simulink model "model_ciagly"  (R2019b)
settings: Solver=FixedStepAuto  StartTime=0  StopTime=4  FixedStep=0.0002  RelTol=1e-3
values from neighbouring files (symbols this model uses):
  J = 22*Js    (= 6.05)    [P.m]    (also in PI.m; faza.m)
  Kp = 1.5*Un/10    (= 33)    [P.m]    (also in PI.m; faza.m)
  Kt = 10/(1.2*wn)    (= 0.0530516476973)    [P.m]    (also in PI.m; faza.m)
  Kw = Mm/(psi_e*kz*Kt*dw*wn)    [P.m]    (also in PI.m = J/(2*Kt*kz*Beta*psi_e); faza.m = J/(2*Kt*kz*Beta*psi_e))
  Mn = psi_e*In    (= 115.854612655)    [P.m]    (also in PI.m; faza.m)
  Rt = 0.15    [P.m]    (also in PI.m; faza.m)
  T = L/R    (= 0.125)    [P.m]    (also in PI.m; faza.m)
  tau0 = 8.1e-3    (= 0.0081)    [P.m]    (also in PI.m; faza.m)
  Y = 10/(2.5*In)    (= 0.0454545454545)    [P.m]    (also in PI.m; faza.m)
undefined symbols (not defined in the file or in its folder): KRi, omega_n, psi_en, Tr_pred, TRi, u_z0
settings Model: Creator=jakub  LastModifiedBy=jakub
settings DataIOCC: SaveFormat=Array

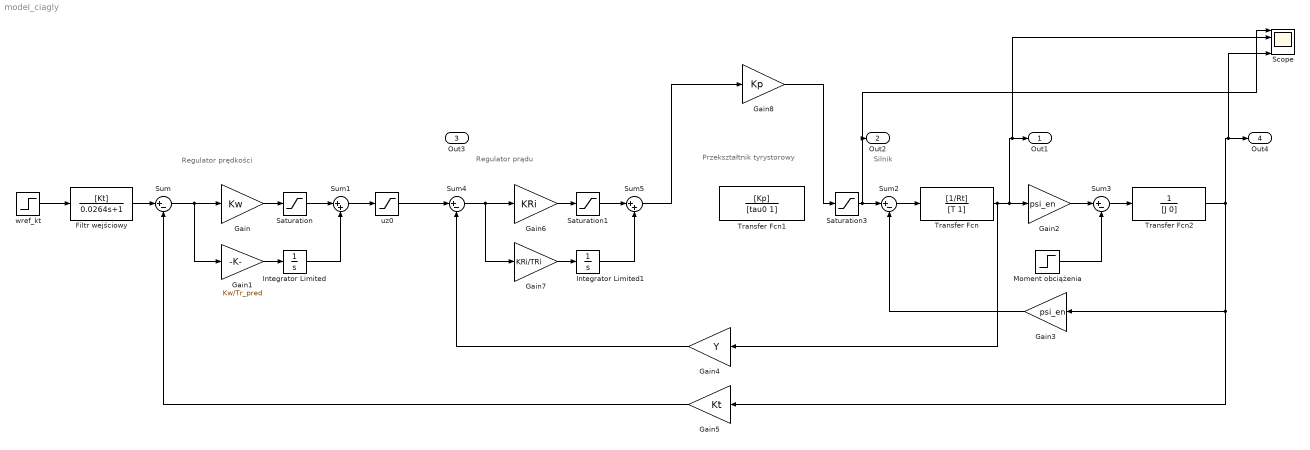
== system model_ciagly ==
  note: Regulator prędkości
  note: Regulator prądu
  note: Przekształtnik
      | tyrystorowy
  note: Silnik
  "Filtr wejściowy " : TransferFcn  Numerator=[Kt]  Denominator=[0.0264 1]
  Gain : Gain  Gain=Kw
  Gain1 : Gain  Gain=Kw/Tr_pred
  Gain2 : Gain  Gain=psi_en
  Gain3 : Gain  Gain=psi_en
  Gain4 : Gain  Gain=Y
  Gain5 : Gain  Gain=Kt
  Gain6 : Gain  Gain=KRi
  Gain7 : Gain  Gain=KRi/TRi
  Gain8 : Gain  Gain=Kp
  Integrator Limited : Integrator  LimitOutput=on  UpperSaturationLimit=10  LowerSaturationLimit=-10
  Integrator Limited1 : Integrator  LimitOutput=on  UpperSaturationLimit=10  LowerSaturationLimit=-10
  Moment obciążenia : Step  Time=0.2  Before=Mn  After=Mn  SampleTime=0
  Saturation : Saturate  UpperLimit=10  LowerLimit=-10
  Saturation1 : Saturate  UpperLimit=10  LowerLimit=-10
  Saturation3 : Saturate  UpperLimit=700  LowerLimit=-700
  Scope : Scope  NumInputPorts=4
  Sum{,2..4} (4 alike) : Sum  Inputs=|+-
  Sum1 : Sum  Inputs=|++
  Sum5 : Sum  Inputs=|++
  Transfer Fcn : TransferFcn  Numerator=[1/Rt]  Denominator=[T 1]
  Transfer Fcn1 : TransferFcn  Numerator=[Kp]  Denominator=[tau0 1]
  Transfer Fcn2 : TransferFcn  Denominator=[J 0]
  uz0 : Saturate  UpperLimit=u_z0  LowerLimit=- u_z0
  "wref_kt " : Step  Time=0  After=omega_n  SampleTime=0
  Out1 : Outport  SignalName=Prad_twornika
  Out2 : Outport  Port=2  SignalName=Napiecie twornika
  Out3 : Outport  Port=3  SignalName=Prad zadany
  Out4 : Outport  Port=4  SignalName=Predkość
  wires:
  "Filtr wejściowy "/1 -> Sum/1
  Sum/1 -> Gain1/1, Gain/1
  Gain1/1 -> Integrator Limited/1
  Integrator Limited/1 -> Sum1/2
  Sum2/1 -> Transfer Fcn/1
  Gain2/1 -> Sum3/1
  Sum3/1 -> Transfer Fcn2/1
  Gain3/1 -> Sum2/2
  Sum4/1 -> Gain7/1, Gain6/1
  Gain7/1 -> Integrator Limited1/1
  Integrator Limited1/1 -> Sum5/2
  Gain4/1 -> Sum4/2
  Gain5/1 -> Sum/2
  Saturation3/1 -> Scope/1, Out2/1, Sum2/1
  Transfer Fcn/1 -> Scope/2, Out1/1, Gain2/1, Gain4/1
  "wref_kt "/1 -> "Filtr wejściowy "/1
  Transfer Fcn2/1 -> Gain5/1, Gain3/1, Scope/4, Out4/1
  Moment obciążenia/1 -> Sum3/2
  Sum1/1 -> uz0/1
  uz0/1 -> Sum4/1
  Gain/1 -> Saturation/1
  Saturation/1 -> Sum1/1
  Saturation1/1 -> Sum5/1
  Gain6/1 -> Saturation1/1
  Sum5/1 -> Gain8/1
  Gain8/1 -> Saturation3/1
